simulink library "Thermosyphon"  (Simulink 8.2)
settings: Solver=ode45  StartTime=0.0  StopTime=10.0  RelTol=1e-3
undefined symbols (not defined in the file): MassFlow, Temperature
libraries: carnot x2, simulink x1, simulink_extras x1
settings Model: Creator=lena.frank  LastModifiedBy=drhf

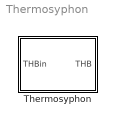
== system Thermosyphon ==
  Thermosyphon : Subsystem  mask(thermosyphon){dia=0.025, fluid_id=water, mix=0, p0=2e5, t1=5}
      mask prompts: dia "diameter at in- and outlet [m]"; fluid_id "fluid"; mix "percentage of fluid mix [0..1]"; p0 "system pressure in [Pa]"; t1 "time constant in s"
      mask help:
      | This block is a model of a "thermosyphon pump". Place it in natural convection systems as you would place a pump.
      | Assure that the sum of heights is zero. Otherwise the simulation will not start.
      | You may check the sum of heights by verifying the "Geodetic Height" in the THB at the inport of this block.
      | If the sum is not zero, the difference is displayed in the subsystem "Stop Simulation".
      mask Help: web(fullfile(path_carnot('help'),'Thermosyphon.html'),'-helpbrowser')
      mask TypeOptions fluid_id: water | air | cotton oil | silicone oil | water-glycol mix | Tyfocor LS
      mask Display:
      | plot(0,0,100,100,[90,10],[80,90],[90,10],[70,80],[90,10],[20,10],[90,10],[30,20],[40,60,40,40],[60,50,40,60])
      | port_label('input',1,'THB')
      | port_label('output',1,'THB')

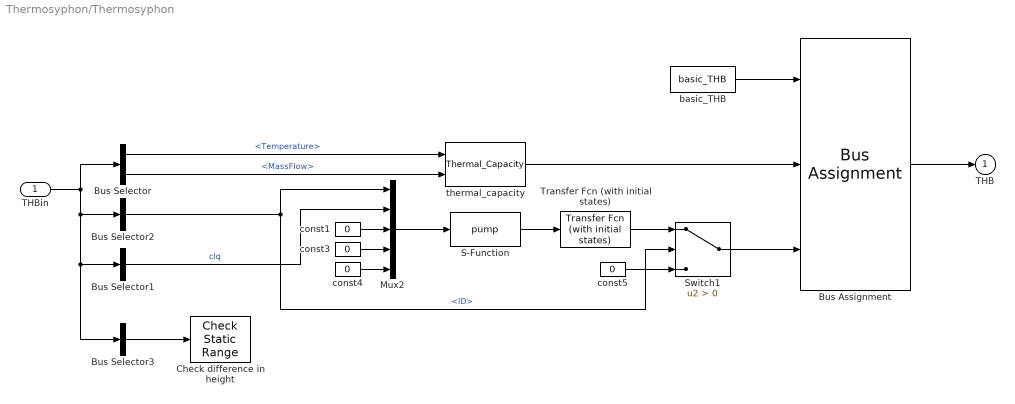
== system Thermosyphon/Thermosyphon ==
  THBin : Inport
  Bus Assignment : BusAssignment  AssignedSignals=Temperature,MassFlow
  Bus Selector : BusSelector  OutputSignals=Temperature,MassFlow
  Bus Selector1 : BusSelector  OutputSignals=DPConstant,DPLinear,DPQuadratic  OutputAsBus=on
  Bus Selector2 : BusSelector  OutputSignals=ID
  Bus Selector3 : BusSelector  OutputSignals=GeodeticHeight  OutputAsBus=on
  Check difference in height : simulink/Model Verification/Check  Static Range  Description=-0.001 <= u <= 0.001  max=0.001  max_included=on  min=-0.001  min_included=on  enabled=on  stopWhenAssertionFail=on  export=off  icon=graphic
  Mux2 : Mux  Inputs=5
  S-Function : S-Function  FunctionName=pump  EnableBusSupport=off
  Switch1 : Switch  Criteria=u2 > Threshold  SaturateOnIntegerOverflow=on  InputSameDT=on
  Transfer Fcn (with initial states) : simulink_extras/Additional Linear/Transfer Fcn (with initial states)  N=[1]  D="[t1  1]"  X0=0
  basic_THB : carnot/Basic/Hydraulics/basic_THB  t=20  mdot=0  p=p0  ID=20001  fluid=fluid_id  mix=mix  dia=dia  hgt=0
  const{1,3..5} (4 alike) : Constant  Value=0
  thermal_capacity : carnot/Basic/Thermal_Models/Thermal_Capacity  UA=1  mcp=t1*100  Tamb=20
  THB : Outport
  wires:
  THBin/1 -> Bus Selector/1, Bus Selector2/1, Bus Selector1/1, Bus Selector3/1
  Bus Selector2/1 -> Mux2/1, Switch1/2  "<ID>"
  Bus Selector/2 -> thermal_capacity/2  "<MassFlow>"
  Bus Selector/1 -> thermal_capacity/1  "<Temperature>"
  Mux2/1 -> S-Function/1
  S-Function/1 -> Transfer Fcn (with initial states)/1
  const3/1 -> Mux2/4
  const4/1 -> Mux2/5
  const1/1 -> Mux2/3
  Transfer Fcn (with initial states)/1 -> Switch1/1
  const5/1 -> Switch1/3
  basic_THB/1 -> Bus Assignment/1
  Bus Assignment/1 -> THB/1
  Bus Selector1/1 -> Mux2/2  "clq"
  thermal_capacity/1 -> Bus Assignment/2
  Switch1/1 -> Bus Assignment/3
  Bus Selector3/1 -> Check difference in height/1
